simulink model "actividad2simulink"  (R2021a)
settings: Solver=VariableStepAuto  StartTime=0.0  StopTime=10.0  RelTol=1e-3
values from neighbouring files (symbols this model uses):
  C = 18e-6    (= 1.8e-05)    [actividad2.m]
  R = 10000    [actividad2.m]
settings Model: Creator=Agus  LastModifiedBy=Agus

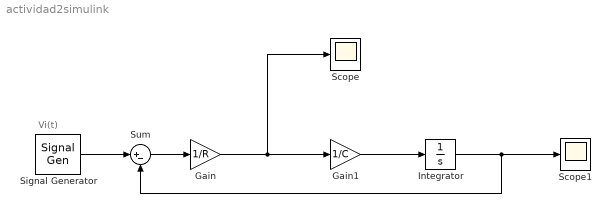
== system actividad2simulink ==
  note: Vi(t)
  Gain : Gain  Gain=1/R
  Gain1 : Gain  Gain=1/C
  Integrator : Integrator
  Scope : Scope
  Scope1 : Scope
  Signal Generator : SignalGenerator
  Sum : Sum  Inputs=|+-
  wires:
  Signal Generator/1 -> Sum/1
  Sum/1 -> Gain/1
  Gain/1 -> Scope/1, Gain1/1
  Gain1/1 -> Integrator/1
  Integrator/1 -> Sum/2, Scope1/1
